simulink model "PlantBandwidth"  (R2025b)
settings: Solver=ode14x  StartTime=0.0  StopTime=10  RelTol=1e-3
model workspace (MAT data in the model file):
  Ki = 200
  Kp = 5000
settings Model: Creator=LYG  LastModifiedBy=mercer

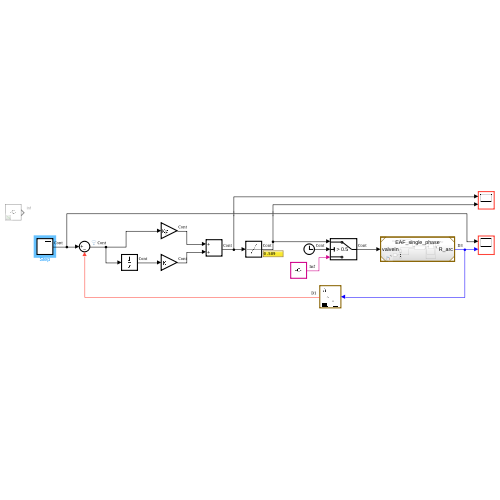
[thumbnail: Simulink's stored preview of the top-level diagram]
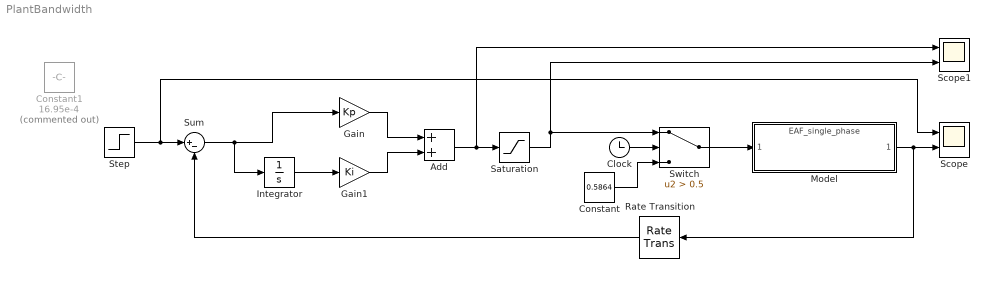
== system PlantBandwidth ==
  Add : Sum
  Clock : Clock
  Constant : Constant  Value=0.5864
  Constant1 : Constant  Commented=on  Value=16.95e-4
  Gain : Gain  Gain=Kp
  Gain1 : Gain  Gain=Ki
  Integrator : Integrator
  Model : ModelReference  ModelNameDialog=EAF_single_phase.slx  SimulationMode=Normal  ModelReferenceVersion=1.22
  Rate Transition : RateTransition
  Saturation : Saturate  UpperLimit=1.2  LowerLimit=-1.2
  Scope : Scope  NumInputPorts=2
      settings: ActiveDisplayYMinimum=-0.0012662091024539378  ActiveDisplayYMaximum=0.011395881922085443
  Scope1 : Scope  NumInputPorts=2
      settings: ActiveDisplayYMinimum=-4.8589834493197337  ActiveDisplayYMaximum=1.4824944415910792
  Step : Step  Time=5  Before=16.95e-4  After=23.95e-4  SampleTime=0
  Sum : Sum  Inputs=|+-
  Switch : Switch  Criteria=u2 > Threshold  Threshold=0.5  SaturateOnIntegerOverflow=off  InputSameDT=off
  wires:
  Gain/1 -> Add/1
  Gain1/1 -> Add/2
  Add/1 -> Scope1/1, Saturation/1
  Integrator/1 -> Gain1/1
  Sum/1 -> Integrator/1, Gain/1
  Model/1 -> Rate Transition/1, Scope/2
  Rate Transition/1 -> Sum/2
  Saturation/1 -> Switch/1, Scope1/2
  Clock/1 -> Switch/2
  Switch/1 -> Model/1
  Constant/1 -> Switch/3
  Step/1 -> Scope/1, Sum/1
